simulink model "blalala"  (R2020b)
settings: Solver=FixedStepAuto  StartTime=0.0  StopTime=0.1
settings Model: Creator=David  LastModifiedBy=marti
settings SolverCC: MaxConsecutiveZCs=100  MaxConsecutiveMinStep=4  ZeroCrossAlgorithm=Adaptive

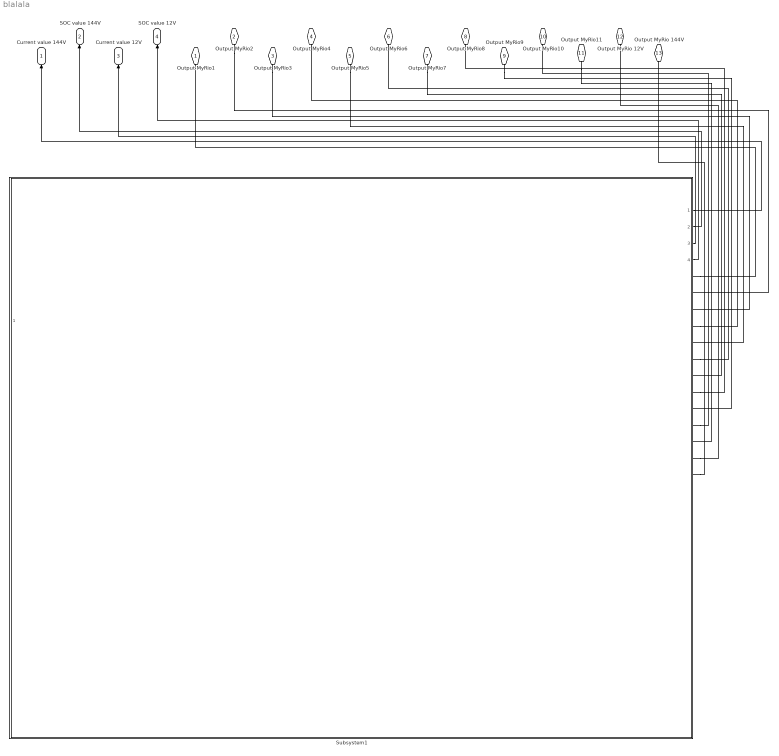
== system blalala ==
  Subsystem1 : Subsystem  ReferencedSubsystem=riktigaBMS
  Output MyRio1 : PMIOPort  Side=Right
  Output MyRio2 : PMIOPort  Port=2  Side=Right
  Output MyRio3 : PMIOPort  Port=3  Side=Right
  Output MyRio4 : PMIOPort  Port=4  Side=Right
  Output MyRio5 : PMIOPort  Port=5  Side=Right
  Output MyRio6 : PMIOPort  Port=6  Side=Right
  Output MyRio7 : PMIOPort  Port=7  Side=Right
  Output MyRio8 : PMIOPort  Port=8  Side=Right
  Output MyRio9 : PMIOPort  Port=9  Side=Right
  Output MyRio10 : PMIOPort  Port=10  Side=Right
  Output MyRio11 : PMIOPort  Port=11  Side=Right
  Output MyRio 12V : PMIOPort  Port=12  Side=Right
  Output MyRio 144V : PMIOPort  Port=13  Side=Right
  Current value 144V : Outport
  SOC value 144V : Outport  Port=2
  Current value 12V : Outport  Port=3
  SOC value 12V : Outport  Port=4
  wires:
  Subsystem1/1 -> Current value 144V/1
  Subsystem1/2 -> SOC value 144V/1
  Subsystem1/3 -> Current value 12V/1
  Subsystem1/4 -> SOC value 12V/1
  connections:
  Subsystem1/RConn1 -- Output MyRio1/RConn1
  Output MyRio2/RConn1 -- Subsystem1/RConn2
  Output MyRio3/RConn1 -- Subsystem1/RConn3
  Subsystem1/RConn4 -- Output MyRio4/RConn1
  Output MyRio5/RConn1 -- Subsystem1/RConn5
  Subsystem1/RConn6 -- Output MyRio6/RConn1
  Output MyRio7/RConn1 -- Subsystem1/RConn7
  Subsystem1/RConn8 -- Output MyRio8/RConn1
  Output MyRio9/RConn1 -- Subsystem1/RConn9
  Subsystem1/RConn10 -- Output MyRio10/RConn1
  Output MyRio11/RConn1 -- Subsystem1/RConn11
  Subsystem1/RConn12 -- Output MyRio 12V/RConn1
  Subsystem1/RConn13 -- Output MyRio 144V/RConn1
